simulink model "PitchControl_FB_linearized"  (R2024b)
settings: Solver=VariableStepAuto  StartTime=0.0  StopTime=150  RelTol=1e-3
libraries: slpidlib x1
settings Model: Creator=Arghya  LastModifiedBy=Arghya

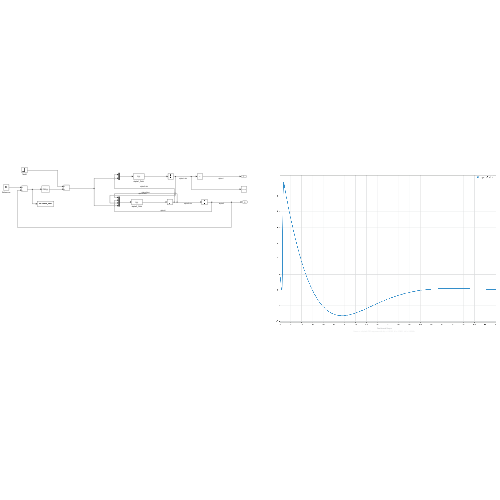
[thumbnail: Simulink's stored preview of the top-level diagram]
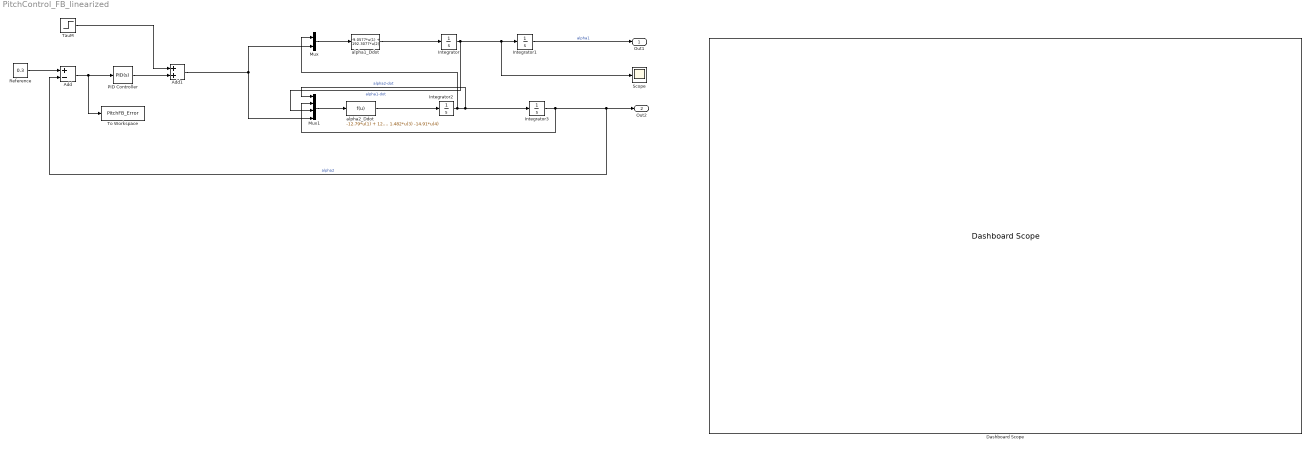
== system PitchControl_FB_linearized ==
  Add : Sum  Inputs=+-
  Add1 : Sum
  Dashboard Scope : DashboardScope  Ymin=0  Ymax=5  LegendPosition=InsideRight
      settings: AttributesFormatString=Name = <Alpha2 PID response with Kp = 0.0153, Ki = 0.0611, Kd = 9.0569>
  Integrator : Integrator  UpperSaturationLimit=pi/2  LowerSaturationLimit=-pi/2  ContinuousStateAttributes="\"alpha1_dot\""
  Integrator1 : Integrator  ContinuousStateAttributes="\"alpha1\""
  Integrator2 : Integrator  UpperSaturationLimit=pi/2  LowerSaturationLimit=-pi/2  ContinuousStateAttributes="\"alpha2_dot\""
  Integrator3 : Integrator  ContinuousStateAttributes="\"alpha2\""
  Mux : Mux  Inputs=2
  Mux1 : Mux
  PID Controller : slpidlib/PID Controller  Controller=PID  Form=Ideal  TimeDomain=Continuous-time  UseExternalTs=off  SampleTime=-1  IntegratorMethod=Forward Euler  FilterMethod=Forward Euler  ControllerParametersSource=internal  P=0.0153319656141861  I=0.0611293239916419  UseKiTs=off  D=9.05683618829529  UseExternalDerivativeSource=off  N=160.157699308039  UseFilter=on  TunerSelectOption=Transfer Function Based (PID Tuner App)  InitialConditionSource=internal  InitialConditionForIntegrator=0  InitialConditionForFilter=0  DifferentiatorICPrevScaledInput=0  ExternalReset=none  TrackingMode=off  Kt=1  LimitOutput=off  SatLimitsSource=internal  UpperSaturationLimit=inf  LowerSaturationLimit=-inf  LinearizeAsGain=on  AntiWindupMode=none  Kb=1  LimitIntegrator=off  UpperIntegratorSaturationLimit=inf  LowerIntegratorSaturationLimit=-inf  POutMin=[]  POutMax=[]  IOutMin=[]  IOutMax=[]  DOutMin=[]  DOutMax=[]  NOutMin=[]  NOutMax=[]  SumOutMin=[]  SumOutMax=[]  SaturationOutMin=[]  SaturationOutMax=[]  PParamMin=[]  PParamMax=[]  IParamMin=[]  IParamMax=[]  DParamMin=[]  DParamMax=[]  NParamMin=[]  NParamMax=[]  KbParamMin=[]  KbParamMax=[]  KtParamMin=[]  KtParamMax=[]  KbOutMin=[]  KbOutMax=[]  KtOutMin=[]  KtOutMax=[]  IntegratorOutMin=[]  IntegratorOutMax=[]  FilterOutMin=[]  FilterOutMax=[]  SumI1OutMin=[]  SumI1OutMax=[]  SumI2OutMin=[]  SumI2OutMax=[]  SumI3OutMin=[]  SumI3OutMax=[]  SumI4OutMin=[]  SumI4OutMax=[]  SumDOutMin=[]  SumDOutMax=[]  DifferentiatorOutMin=[]  DifferentiatorOutMax=[]  FilterDiffOutCoefMin=[]  FilterDiffOutCoefMax=[]  ReciprocalOutMin=[]  ReciprocalOutMax=[]  SumDenOutMin=[]  SumDenOutMax=[]  SumNumOutMin=[]  SumNumOutMax=[]  DivideOutMin=[]  DivideOutMax=[]  UdiffTsProdOutMin=[]  UdiffTsProdOutMax=[]  NTsProdOutMin=[]  NTsProdOutMax=[]  UintegralTsProdOutMin=[]  UintegralTsProdOutMax=[]  UngainTsProdOutMin=[]  UngainTsProdOutMax=[]  ClampingZeroOutDataTypeStr=Inherit: Inherit via back propagation  ClampingZeroOutMin=[]  ClampingZeroOutMax=[]  FilterDenConstantOutDataTypeStr=Inherit: Inherit via back propagation  FilterDenConstantOutMin=[]  FilterDenConstantOutMax=[]  PCopyOutDataTypeStr=Inherit: Inherit via back propagation  PCopyOutMin=[]  PCopyOutMax=[]  NCopyOutDataTypeStr=Inherit: Inherit via back propagation  NCopyOutMin=[]  NCopyOutMax=[]  IntegratorContinuousStateAttributes=''  IntegratorStateMustResolveToSignalObject=off  IntegratorRTWStateStorageClass=Auto  FilterContinuousStateAttributes=''  FilterStateMustResolveToSignalObject=off  FilterRTWStateStorageClass=Auto  ParallelPVariant=Passthrough  IdealPVariant=InternalParameters  IVariant=InternalParameters  DVariant=InternalParameters  IntegratorVariant=Continuous  SatVariant=Disabled  AWVariant=Passthrough  PCopyVariant=Disabled  TRVariant=Disabled  FdbkBlocksVariant=Forward  IdealPFdbkVariant=Disabled  SatFdbkVariant=Disabled  DerivativeFilterVariant=ContFilter  NVariant=InternalParameters  NCopyVariant=Disabled  FilterICVariant=InternalICsFilter  IntegratorICVariant=InternalICs  ExternalResetVariant=Disabled  TRSumVariant=Passthrough  SumFdbkVariant=Disabled  SumVariant=Sum_PID  TsampFilterVariant=InternalTs  TsampNgainVariant=Passthrough  TsampIntegralVariant=Disabled_SignalSpec  ExternalSaturationOutDataTypeStr=Inherit: Same as second input  DerivativeSourceVariant=ErrorSignal  PreIntVariant=InternalPreInt
  Reference : Constant  Value=0.3
  Scope : Scope
  TauM : Step  SampleTime=0
  To Workspace : ToWorkspace  VariableName=PitchFB_Error  SampleTime=-1
  alpha1_Ddot : Fcn  Expr=-9.0577*u(1) + 192.3077*u(2)
  alpha2_Ddot : Fcn  Expr=-12.79*u(1) + 12.2*u(2) + 1.482*u(3) -14.91*u(4)
  Out1 : Outport
  Out2 : Outport  Port=2
  wires:
  Integrator/1 -> Mux1/3, Scope/1, Integrator1/1  "alpha1-dot"
  Integrator2/1 -> Mux1/1, Integrator3/1, Mux/1  "alpha2-dot"
  alpha2_Ddot/1 -> Integrator2/1
  alpha1_Ddot/1 -> Integrator/1
  Integrator1/1 -> Out1/1  "alpha1"
  Integrator3/1 -> Mux1/2, Add/2, Out2/1  "alpha2"
  Mux/1 -> alpha1_Ddot/1
  Mux1/1 -> alpha2_Ddot/1
  Reference/1 -> Add/1
  Add1/1 -> Mux1/4, Mux/2
  TauM/1 -> Add1/1
  PID Controller/1 -> Add1/2
  Add/1 -> PID Controller/1, To Workspace/1
